simulink model "AModelS"  (R2020b)
settings: Solver=VariableStepAuto  StartTime=0.0  StopTime=10.0  RelTol=1e-3
values from neighbouring files (symbols this model uses):
  DES_POS = [pi/2,0]    [Alternative_Init.m]    (also in init.m)
  INITIAL_CONDITIONS = [0,0,0,0]    [Alternative_Init.m]    (also in init.m = [-pi/2,0,0,0]; lqr_init.m = [pi + pi/12, -pi/12, 0, 0])
  PARAM = [m1,m2,I1,lc1,l2,lc2,I1,I2]    [Alternative_Init.m]    (also in init.m)
settings Model: Creator=gianl  LastModifiedBy=gianl

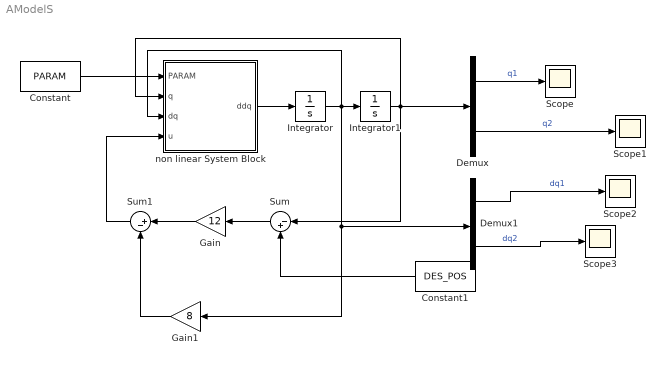
== system AModelS ==
  Constant : Constant  Value=PARAM
  Constant1 : Constant  Value=DES_POS
  Demux : Demux  Outputs=2
  Demux1 : Demux  Outputs=2
  Gain : Gain  Gain=12
  Gain1 : Gain  Gain=8
  Integrator : Integrator  InitialCondition=INITIAL_CONDITIONS(2:3)
  Integrator1 : Integrator  InitialCondition=INITIAL_CONDITIONS(1:2)
  Scope{,1..3} (4 alike) : Scope
  Sum : Sum  Inputs=|-+
  Sum1 : Sum  Inputs=|+-
  non linear System Block : MATLAB Function  TreatAsAtomicUnit=on
  wires:
  Demux/1 -> Scope/1  "q1"
  Demux/2 -> Scope1/1  "q2"
  Demux1/2 -> Scope3/1  "dq2"
  non linear System Block/1(ddq) -> Integrator/1
  Demux1/1 -> Scope2/1  "dq1"
  Integrator1/1 -> Sum/1, non linear System Block/2(q), Demux/1
  Constant/1 -> non linear System Block/1(PARAM)
  Sum/1 -> Gain/1
  Constant1/1 -> Sum/2
  Gain/1 -> Sum1/1
  Gain1/1 -> Sum1/2
  Integrator/1 -> Gain1/1, Demux1/1, non linear System Block/3(dq), Integrator1/1
  Sum1/1 -> non linear System Block/4(u)

== matlab function AModelS/non linear System Block ==
  data: PARAM input; q input size=2; dq input size=2; u input size=2; ddq output size=2
function ddq = nonlinearSys(PARAM,q,dq,u)
m1 = PARAM(1);              % giunto 1 mass
m2 = PARAM(2);              % giunto 2 mass
l1 = PARAM(3);          % lunghezza primo giunto
lc1 = PARAM(4);          % centro di massa giunto 1
l2 = PARAM(5);
lc2 = PARAM(6);
I1 = PARAM(7);
I2 = PARAM(8);
g= 9.81;

q1 = q(1);
q2 = q(2);
dq1 = dq(1);
dq2= dq(2);

% M =[  1.25*cos(q2) + 1.875, 0.625*cos(q2) + 0.3125;
%     0.625*cos(q2) + 0.3125,                 0.3125];
% 
% C =[- (5*dq1*dq2*sin(q2))/8 - (5*dq2*sin(q2)*(dq1 + dq2))/8;
%                                     (5*dq1^2*sin(q2))/8];
%  
% G =[ - (49*cos(q1 + q2))/4 - (147*cos(q1))/4;
%        -(49*cos(q1 + q2))/4];
% n= C+G;
%    
a1 = I1+ I2+ m1*lc1^2+m2*(l1^2+lc2^2);
a2 = m2*l1*lc2^2;
a3 = I2 + m2*lc2^2;
a4 = g*(m1*lc1+m2*l1);
a5 = g*m2*lc2;

M = [a1+2*a2*cos(q2), a3+a2*cos(q2);
     a3+a2*cos(q2), a3];
 
c = [-a2*dq2*(dq2+2*dq1)*sin(q2);
    a2*dq1^2*sin(q2)];
e = [ a4*cos(q1) + a5*cos(q1+q2);
    a5*cos(q1+q2)];
n = c+e;
ddq =M\(u-n);
